simulink model "s4"  (R2016b)
settings: Solver=VariableStepAuto  StartTime=0.0  StopTime=10.0  RelTol=1e-3
settings Model: Creator=fabia  LastModifiedBy=fabia

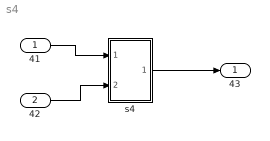
== system s4 ==
  41 : Inport
  42 : Inport  Port=2
  s4 : Subsystem
  43 : Outport
  wires:
  41/1 -> s4/1(In1)
  42/1 -> s4/2(In2)
  s4/1(Out1) -> 43/1

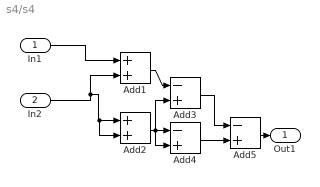
== system s4/s4 ==
  In1 : Inport
  In2 : Inport  Port=2
  Add1 : Sum
  Add2 : Sum
  Add3 : Sum  Inputs=-+
  Add4 : Sum  Inputs=-+
  Add5 : Sum  Inputs=-+
  Out1 : Outport
  wires:
  In1/1 -> Add1/1
  In2/1 -> Add2/2, Add2/1, Add1/2
  Add1/1 -> Add3/1
  Add4/1 -> Add5/2
  Add5/1 -> Out1/1
  Add3/1 -> Add5/1
  Add2/1 -> Add3/2, Add4/1, Add4/2
